simulink model "B"  (R2022b)
settings: Solver=VariableStepAuto  StartTime=0.0  StopTime=10.0  RelTol=1e-3
settings Model: Creator=LYZ  LastModifiedBy=LYZ

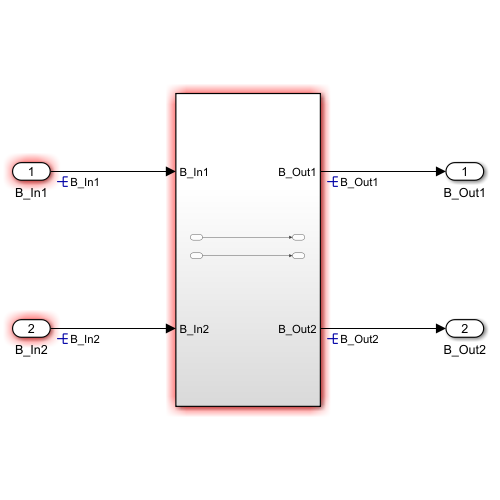
[thumbnail: Simulink's stored preview of the top-level diagram]
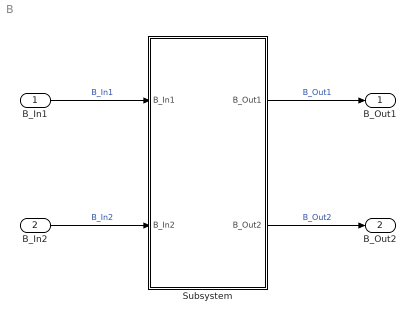
== system B ==
  B_In1 : Inport
  B_In2 : Inport  Port=2
  Subsystem : Subsystem
  B_Out1 : Outport
  B_Out2 : Outport  Port=2
  wires:
  Subsystem/1(B_Out1) -> B_Out1/1  "B_Out1"
  B_In2/1 -> Subsystem/2(B_In2)  "B_In2"
  B_In1/1 -> Subsystem/1(B_In1)  "B_In1"
  Subsystem/2(B_Out2) -> B_Out2/1  "B_Out2"

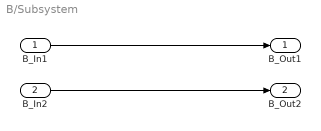
== system B/Subsystem ==
  B_In1 : Inport
  B_In2 : Inport  Port=2
  B_Out1 : Outport
  B_Out2 : Outport  Port=2
  wires:
  B_In1/1 -> B_Out1/1
  B_In2/1 -> B_Out2/1
